simulink model "RLBicycleSimulinkP2P"  (R2021a)
settings: Solver=VariableStepAuto  StartTime=0.0  StopTime=500  RelTol=1e-3
model workspace (MAT data in the model file):
  Sig = Simulink.Signal
  Sig.DataType = 'auto'
  Sig.Dimensions = -1
  Sig.DimensionsMode = 'auto'
  Sig.Complexity = 'auto'
  Sig.SampleTime = -1
  Sig.SamplingMode = 'auto'
undefined symbols (not defined in the file or in its folder): chosenMap, distMax, distMin, goalPose, speedMax, startPose, steeringRange
libraries: simulink x2, rllib x1
settings Model: OrderedModelArguments=off  Creator=The MathWorks, Inc.  LastModifiedBy=guyot
settings SolverCC: AlgebraicLoopSolver=TrustRegion
settings DebuggingCC: SymbolicDimsDataTypeCodeGenerationDiagnostic=none  SFMachineParentedDataDiag=warning

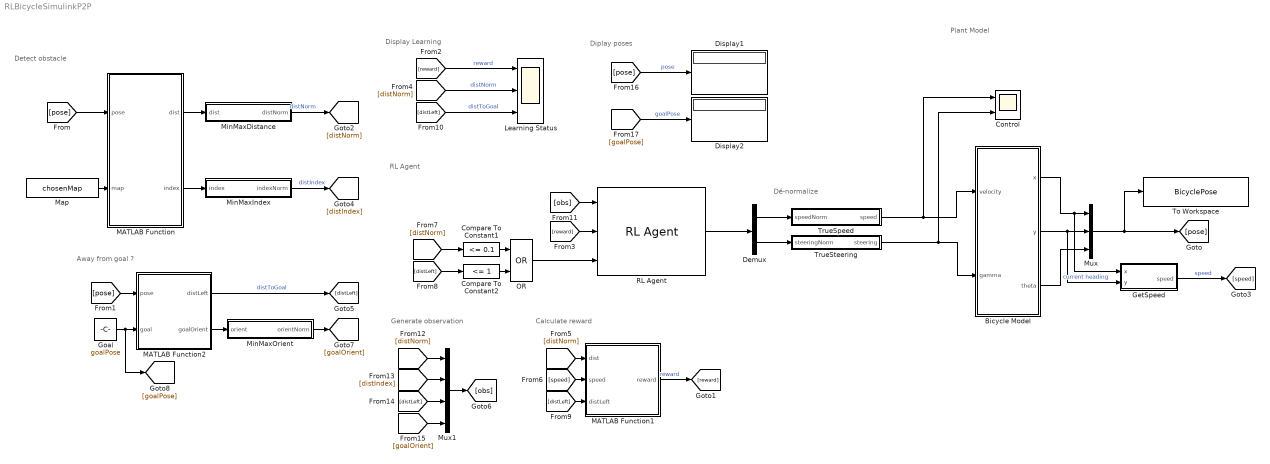
== system RLBicycleSimulinkP2P ==
  note: Diplay poses
  note: Calculate reward
  note: Generate observation
  note: Away from goal ?
  note: Detect obstacle
  note: Display Learning
  note: RL Agent
  note: Dé-normalize
  note: Plant Model
  Bicycle Model : Subsystem
  Compare To Constant1 : simulink/Logic and Bit Operations/Compare To Constant  relop=<=  const=0.1  OutDataTypeStr=boolean
  Compare To Constant2 : simulink/Logic and Bit Operations/Compare To Constant  relop=<=  const=1  OutDataTypeStr=boolean
  Control : Scope  NumInputPorts=2
  Demux : Demux  Outputs=2
  Display1 : Display
  Display2 : Display
  GetSpeed : Subsystem
  Goal : Constant  Value=goalPose
  Learning Status : Scope  NumInputPorts=3
  MATLAB Function : MATLAB Function  TreatAsAtomicUnit=on
  MATLAB Function1 : MATLAB Function  TreatAsAtomicUnit=on
  MATLAB Function2 : MATLAB Function  TreatAsAtomicUnit=on
  Map : Constant  Value=chosenMap
  MinMaxDistance : Subsystem
  MinMaxIndex : Subsystem
  MinMaxOrient : Subsystem
  Mux : Mux  Inputs=3
  Mux1 : Mux
  OR : Logic  Operator=OR  IconShape=distinctive  AllPortsSameDT=off  OutDataTypeStr=boolean
  RL Agent : rllib/RL Agent  Agent=agent  ExternalActionAsInput=off  ProvideCumRwd=off  TreatAsDirectFeedthrough=on
  To Workspace : ToWorkspace  VariableName=BicyclePose  SampleTime=-1
  TrueSpeed : Subsystem
  TrueSteering : Subsystem
  wires:
  Map/1 -> MATLAB Function/2(map)
  Mux/1 -> To Workspace/1, [pose]
  RL Agent/1 -> Demux/1
  MATLAB Function1/1(reward) -> [reward]  "reward"
  Bicycle Model/3(theta) -> Mux/3  "current heading"
  Bicycle Model/2(y) -> GetSpeed/2(y), Mux/2
  Bicycle Model/1(x) -> GetSpeed/1(x), Mux/1
  MATLAB Function/1(dist) -> MinMaxDistance/1(dist)
  TrueSpeed/1(speed) -> Bicycle Model/1(velocity), Control/1
  Demux/2 -> TrueSteering/1(steeringNorm)
  TrueSteering/1(steering) -> Bicycle Model/2(gamma), Control/2
  Demux/1 -> TrueSpeed/1(speedNorm)
  [obs] -> RL Agent/1
  MATLAB Function/2(index) -> MinMaxIndex/1(index)
  Goal/1 -> [goalPose], MATLAB Function2/2(goal)
  Compare To Constant1/1 -> OR/1
  Compare To Constant2/1 -> OR/2
  OR/1 -> RL Agent/3
  [pose] -> MATLAB Function/1(pose)
  [pose] -> MATLAB Function2/1(pose)
  [reward] -> Learning Status/1  "reward"
  [reward] -> RL Agent/2
  MinMaxDistance/1(distNorm) -> [distNorm]  "distNorm"
  [distNorm] -> Learning Status/2  "distNorm"
  [distNorm] -> MATLAB Function1/1(dist)
  GetSpeed/1(speed) -> [speed]  "speed"
  [speed] -> MATLAB Function1/2(speed)
  [distNorm] -> Compare To Constant1/1
  MinMaxIndex/1(indexNorm) -> [distIndex]  "distIndex"
  MATLAB Function2/1(distLeft) -> [distLeft]  "distToGoal"
  [distLeft] -> Compare To Constant2/1
  [distLeft] -> MATLAB Function1/3(distLeft)
  [distLeft] -> Learning Status/3  "distToGoal"
  Mux1/1 -> [obs]
  [distNorm] -> Mux1/1
  [distIndex] -> Mux1/2
  [distLeft] -> Mux1/3
  [goalOrient] -> Mux1/4
  MinMaxOrient/1(orientNorm) -> [goalOrient]
  MATLAB Function2/2(goalOrient) -> MinMaxOrient/1(orient)
  [pose] -> Display1/1  "pose"
  [goalPose] -> Display2/1  "goalPose"

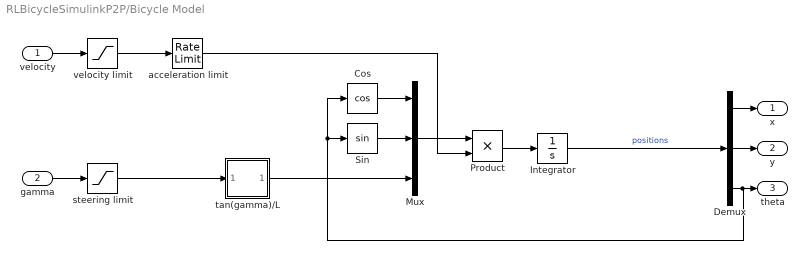
== system RLBicycleSimulinkP2P/Bicycle Model ==
  velocity : Inport
  gamma : Inport  Port=2
  Cos : Trigonometry  Operator=cos
  Demux : Demux  Outputs=3
  Integrator : Integrator  InitialCondition=startPose
  Mux : Mux  Inputs=3
  Product : Product
  Sin : Trigonometry
  acceleration limit : RateLimiter  RisingSlewLimit=0.2  SampleTimeMode=inherited
  steering limit : Saturate  UpperLimit=steeringRange  LowerLimit=-steeringRange
  tan(gamma)/L : Subsystem
  velocity limit : Saturate  UpperLimit=speedMax  LowerLimit=-speedMax
  x : Outport
  y : Outport  Port=2
  theta : Outport  Port=3
  wires:
  velocity/1 -> velocity limit/1
  velocity limit/1 -> acceleration limit/1
  gamma/1 -> steering limit/1
  steering limit/1 -> tan(gamma)/L/1(In1)
  tan(gamma)/L/1(Out1) -> Mux/3
  Mux/1 -> Product/1
  acceleration limit/1 -> Product/2
  Product/1 -> Integrator/1
  Integrator/1 -> Demux/1  "positions"
  Demux/3 -> Cos/1, Sin/1, theta/1
  Demux/1 -> x/1
  Demux/2 -> y/1
  Cos/1 -> Mux/1
  Sin/1 -> Mux/2

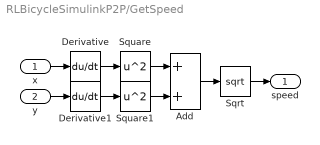
== system RLBicycleSimulinkP2P/GetSpeed ==
  x : Inport
  y : Inport  Port=2
  Add : Sum
  Derivative : Derivative
  Derivative1 : Derivative
  Sqrt : Sqrt  SaturateOnIntegerOverflow=on
  Square : Math  Operator=square  SaturateOnIntegerOverflow=on
  Square1 : Math  Operator=square  SaturateOnIntegerOverflow=on
  speed : Outport
  wires:
  Derivative/1 -> Square/1
  Add/1 -> Sqrt/1
  Square/1 -> Add/1
  x/1 -> Derivative/1
  y/1 -> Derivative1/1
  Derivative1/1 -> Square1/1
  Square1/1 -> Add/2
  Sqrt/1 -> speed/1

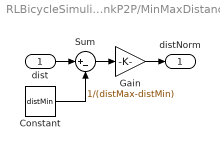
== system RLBicycleSimulinkP2P/MinMaxDistance ==
  dist : Inport
  Constant : Constant  Value=distMin
  Gain : Gain  Gain=1/(distMax-distMin)
  Sum : Sum  Inputs=|+-
  distNorm : Outport
  wires:
  Constant/1 -> Sum/2
  Sum/1 -> Gain/1
  dist/1 -> Sum/1
  Gain/1 -> distNorm/1

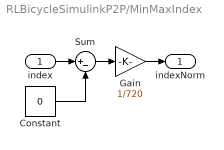
== system RLBicycleSimulinkP2P/MinMaxIndex ==
  index : Inport
  Constant : Constant  Value=0
  Gain : Gain  Gain=1/720
  Sum : Sum  Inputs=|+-
  indexNorm : Outport
  wires:
  Constant/1 -> Sum/2
  Sum/1 -> Gain/1
  index/1 -> Sum/1
  Gain/1 -> indexNorm/1

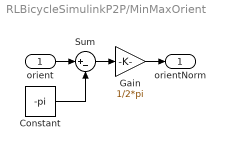
== system RLBicycleSimulinkP2P/MinMaxOrient ==
  orient : Inport
  Constant : Constant  Value=-pi
  Gain : Gain  Gain=1/2*pi
  Sum : Sum  Inputs=|+-
  orientNorm : Outport
  wires:
  Constant/1 -> Sum/2
  Sum/1 -> Gain/1
  orient/1 -> Sum/1
  Gain/1 -> orientNorm/1

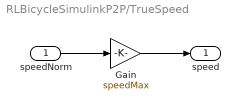
== system RLBicycleSimulinkP2P/TrueSpeed ==
  speedNorm : Inport
  Gain : Gain  Gain=speedMax
  speed : Outport
  wires:
  Gain/1 -> speed/1
  speedNorm/1 -> Gain/1

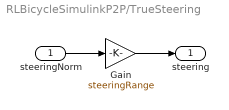
== system RLBicycleSimulinkP2P/TrueSteering ==
  steeringNorm : Inport
  Gain : Gain  Gain=steeringRange
  steering : Outport
  wires:
  steeringNorm/1 -> Gain/1
  Gain/1 -> steering/1

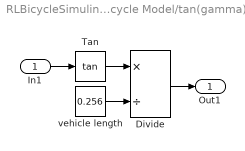
== system RLBicycleSimulinkP2P/Bicycle Model/tan(gamma)//L ==
  In1 : Inport
  Divide : Product  Inputs=*/
  Tan : Trigonometry  Operator=tan
  vehicle length : Constant  Value=0.256
  Out1 : Outport
  wires:
  Tan/1 -> Divide/1
  vehicle length/1 -> Divide/2
  In1/1 -> Tan/1
  Divide/1 -> Out1/1

== matlab function RLBicycleSimulinkP2P/MATLAB Function1 ==
  data: dist input; reward output; speed input; distLeft input
function reward = calcRew(dist, speed, distLeft)
    % Fonction de calcul de recompense
    % coefficients a tuner
    if distLeft <= 1.1
        reward = 15;
    elseif dist < 0.1
        % Touche un mur : punition
        reward = -10;
    elseif dist < 0.3
        % Proche d'un mur : tout faire pour le pas le toucher quelle que
        % soit la vitesse
        reward = dist;
    else
        % Loin d'un mur : maximiser la vitesse en privilégiant avancée
        reward = dist + 5*speed + 5/distLeft;
    end

== matlab function RLBicycleSimulinkP2P/MATLAB Function ==
  data: pose input; map input; dist output; index output
function [dist, index]  = distMin(pose, map)
    % Trouve la distance minimale dans un cône devant le véhicule
    % alpha : angle du cône
    binaryMap = binaryOccupancyMap(map);
    maxrange = 3;
    angles = [];
    step = deg2rad(0.5);
    
    % Le LIDAR de la Qcar a une détection d'objets à 360° tous les 0.5°
    for i = 0:step:2*pi-step
        angles = [angles i]; % 720 points
    end
    
    intsectionPts = rayIntersection(binaryMap,pose,angles,maxrange);
    
    % Recherche de la distance minimale à l'avant
    intsectionRelative = [intsectionPts(:,1)-pose(1) intsectionPts(:,2)-pose(2)];
    intsectionDist = sqrt(intsectionRelative(:,1).^2 + intsectionRelative(:,2).^2);
    [dist, index] = min(intsectionDist,[],1,'linear');
    if isnan(dist)
        dist = 5;
        index = 0;
    end

== matlab function RLBicycleSimulinkP2P/MATLAB Function2 ==
  data: pose input; distLeft output; goal input; goalOrient output
function [distLeft,goalOrient] = euclidDist(pose, goal)
    relativePose = goal - pose;

distLeft = sqrt(relativePose(1).^2+relativePose(2).^2);
goalOrient = atan2(relativePose(2),relativePose(1));
